simulink model "aquecedor_2_partes"  (Simulink 7.9)
settings: Solver=ode45  StartTime=0.0  StopTime=4000  RelTol=1e-3
values from neighbouring files (symbols this model uses):
  C1 = V1*water_density*water_specific_heat    (= 525000)    [aquecedor_2_partes.m]
  C2 = V2*air_density*air_specific_heat    (= 130)    [aquecedor_2_partes.m]
  qe = 1000    [aquecedor_2_partes.m]
  R1 = W1 / (COND1 * A)    (= 0.001)    [aquecedor_2_partes.m]
  R2 = W2 / (COND2 * A)    (= 0.00025974025974)    [aquecedor_2_partes.m]
  Te = 20    [aquecedor_2_partes.m]
settings Model: Creator=paulo.costa  LastModifiedBy=paulo.costa

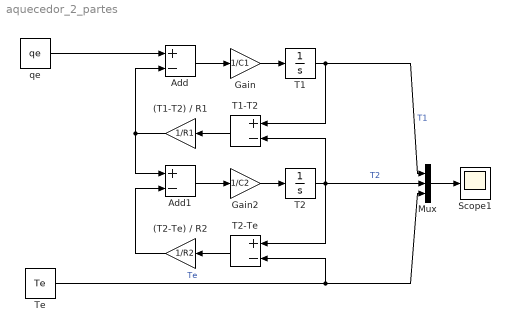
== system aquecedor_2_partes ==
  (T1-T2) / R1 : Gain  Gain=1/R1
  (T2-Te) / R2 : Gain  Gain=1/R2
  Add : Sum  Inputs=+-
  Add1 : Sum  Inputs=+-
  Gain : Gain  Gain=1/C1
  Gain2 : Gain  Gain=1/C2
  Mux : Mux  Inputs=3
  Scope1 : Scope
  T1 : Integrator  InitialCondition=Te
  T1-T2 : Sum  Inputs=+-
  T2 : Integrator  InitialCondition=Te
  T2-Te : Sum  Inputs=+-
  Te : Constant  Value=Te
  qe : Constant  Value=qe
  wires:
  qe/1 -> Add/1
  Gain/1 -> T1/1
  Add/1 -> Gain/1
  T1/1 -> T1-T2/1, Mux/1  "T1"
  (T1-T2) / R1/1 -> Add/2, Add1/1
  T1-T2/1 -> (T1-T2) / R1/1
  Gain2/1 -> T2/1
  Add1/1 -> Gain2/1
  T2/1 -> T2-Te/1, T1-T2/2, Mux/2  "T2"
  (T2-Te) / R2/1 -> Add1/2
  T2-Te/1 -> (T2-Te) / R2/1
  Te/1 -> T2-Te/2, Mux/3  "Te"
  Mux/1 -> Scope1/1
